simulink model "BMVModel"  (R2020a)
settings: Solver=VariableStepAuto  StartTime=0.0  StopTime=10.0  RelTol=1e-3
values from neighbouring files (symbols this model uses):
  BMV_Spring_Constant = spring_constant    [run_monte_carlo.m]
undefined symbols (not defined in the file or in its folder): Displacement, Pressure
libraries: BrakeSystemLibrary x1
settings Model: Creator=Jared  LastModifiedBy=Jared

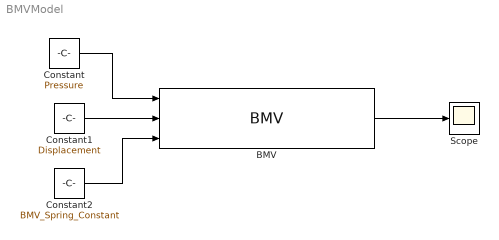
== system BMVModel ==
  BMV : BrakeSystemLibrary/Brake System/BMV  SystemSampleTime=-1  Latency=0  AutoFrameSizeCalculation=off
  Constant : Constant  Value=Pressure
  Constant1 : Constant  Value=Displacement
  Constant2 : Constant  Value=BMV_Spring_Constant
  Scope : Scope
  wires:
  Constant/1 -> BMV/1
  Constant1/1 -> BMV/2
  Constant2/1 -> BMV/3
  BMV/1 -> Scope/1
